simulink model "Adaptive_BS_jointspace"  (R2021b)
settings: Solver=VariableStepAuto  StartTime=0.0  StopTime=15.0  RelTol=1e1
undefined symbols (not defined in the file): Kd, l1, l2, l3, l4, l5, l6, lambda, m1, m2, m3, m4, m5, m6, q0, r
libraries: roblocks x3
(part 5 of 5)

== matlab function Adaptive_BS_jointspace/ABS control/parameters estimation ==
  data: Y input; dpi output; s input
function dpi = dyn_param(Y, s)
% Definisco una matrice definita positiva
R = 5*diag([0.1 11 25 54 55 298]);
% Calcolo la dinamica di stima dei parametri
dpi = inv(R) * Y' * s;
